simulink model "RoboCupManipulation_Simulink_ROS_Control"  (R2020b)
settings: Solver=FixedStepAuto  StartTime=0.0  StopTime=15  FixedStep=0.1  RelTol=1e-3
PreLoadFcn:
  | load('exampleHelperKINOVAGen3GripperROSGazebo.mat');
model workspace (MAT data in the model file):
  SL_ROS_VariableLengthArrays_MaxSizes.CommonInfo.ArrayTruncateAction = 'EmitWarning'
  SL_ROS_VariableLengthArrays_MaxSizes.MsgTypeMap = containers.Map
  SL_ROS_VariableLengthArrays_MaxSizes.MsgTypeMap.serialization.keys = {'sensor_msgs/Image'}
  SL_ROS_VariableLengthArrays_MaxSizes.MsgTypeMap.serialization.values{1}(1).PropertyName = 'Data'
  SL_ROS_VariableLengthArrays_MaxSizes.MsgTypeMap.serialization.values{1}(1).DataType = 'uint8'
  SL_ROS_VariableLengthArrays_MaxSizes.MsgTypeMap.serialization.values{1}(1).MaxLength = 518400
  SL_ROS_VariableLengthArrays_MaxSizes.MsgTypeMap.serialization.values{1}(2).PropertyName = 'Encoding'
  SL_ROS_VariableLengthArrays_MaxSizes.MsgTypeMap.serialization.values{1}(2).DataType = 'uint8'
  SL_ROS_VariableLengthArrays_MaxSizes.MsgTypeMap.serialization.values{1}(2).MaxLength = 128
  SL_ROS_VariableLengthArrays_MaxSizes.MsgTypeMap.serialization.uniformity = 0
  SL_ROS_VariableLengthArrays_MaxSizes.MsgTypeMap.serialization.keyType = 'char'
  SL_ROS_VariableLengthArrays_MaxSizes.MsgTypeMap.serialization.valueType = 'any'
undefined symbols (not defined in the file or in its folder): Angle, Axis, eul2tform, trvec2tform
libraries: robotlib x7, robotcorelib x5, robotmaniplib x2, robotgazebolib x1, simulink x1
settings Model: PacingRate=0.220000  Creator=amavromm  LastModifiedBy=josea
settings OptimizationCC: EnhancedBackFolding=on  PassReuseOutputArgsAs=Individual arguments  ZeroExternalMemoryAtStartup=off  ZeroInternalMemoryAtStartup=off  MaxStackSize=64  OptimizeBlockOrder=speed  DifferentSizesBufferReuse=on  OptimizationCustomize=off  EfficientTunableParamExpr=on
settings DebuggingCC: ParameterTunabilityLossMsg=error
settings HardwareCC: ProdBitPerPointer=32  ProdBitPerSizeT=32  ProdBitPerPtrDiffT=32  ProdLargestAtomicFloat=None  ProdIntDivRoundTo=Undefined  ProdEndianess=Unspecified  ProdWordSize=32  ProdHWDeviceType=Generic->Unspecified (assume 32-bit Generic)
settings SFSimCC: MATLABDynamicMemAlloc=off  SimTargetLang=C++
settings RTWCC: Description=Embedded Coder  SystemTargetFile=ert.tlc  HardwareBoard=Robot Operating System (ROS)  TLCOptions="-aInlineSetEventsForThisBaseRateFcn=TLC_FALSE -aSuppressMultiTaskScheduler=TLC_FALSE  -aRateBasedStepFcn=0"  TemplateMakefile=ert_default_tmf  Toolchain=Catkin  TargetLang=C++
settings CodeAppCC: ForceParamTrailComments=on  IgnoreCustomStorageClasses=off  OperatorAnnotations=on  SimulinkDataObjDesc=on  SFDataObjDesc=on  InsertBlockDesc=on

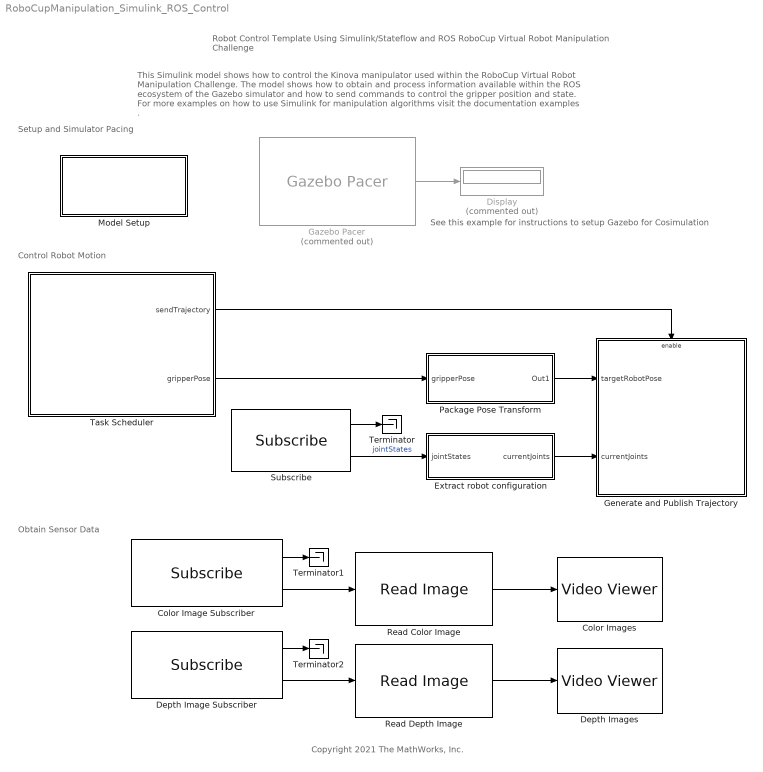
== system RoboCupManipulation_Simulink_ROS_Control ==
  note: See this example for instructions to setup Gazebo for Cosimulation
  note: This Simulink model shows how to control the Kinova manipulator used within the RoboCup Virtual Robot Manipulation Challenge. The model shows how to obtain and process information available within the ROS ecosystem of the Gazebo simulator and how to send commands to control the gripper position and state. For more examples on how to use Simulink for manipulation algorithms visit the documentation examples .
  note: Robot Control Template Using Simulink/Stateflow and ROS
      | RoboCup Virtual Robot Manipulation Challenge
  note: Obtain Sensor Data
  note: Control Robot Motion
  note: Setup and Simulator Pacing
  note: Copyright 2021 The MathWorks, Inc.
  Color Image Subscriber : robotlib/Subscribe  topicSource=Select from ROS network  topic=/camera/color/image_raw  messageType=sensor_msgs/Image  SampleTime=0.5  legacyBusStruct=off  messageQueueLength=1
  Color Images : VideoViewer  FigPos=[757 790 418 304]
  Depth Image Subscriber : robotlib/Subscribe  topicSource=Select from ROS network  topic=/camera/depth/image_raw  messageType=sensor_msgs/Image  SampleTime=0.5  legacyBusStruct=off  messageQueueLength=1
  Depth Images : VideoViewer  FigPos=[241 742 418 304]
  Display : Display  Commented=on
  Extract robot configuration : Subsystem
  Gazebo Pacer : robotgazebolib/Gazebo Pacer  Commented=on  ResetBehavior=Reset Gazebo simulation time  SampleTime=0.1
      settings: SourceProductBaseCode=RO
  Generate and Publish Trajectory : Subsystem
  Model Setup : Subsystem
  Package Pose Transform : Subsystem
  Read Color Image : robotlib/Read Image  MaximumImageSize=[270, 480]  ImageEncoding=rgb8  ShowAlphaOutput=off  ShowErrorCodeOutput=off  VariableSizeOutputs=off
      settings: SourceProductBaseCode=RR
  Read Depth Image : robotlib/Read Image  MaximumImageSize=[270, 480]  ImageEncoding=32fc1  ShowAlphaOutput=off  ShowErrorCodeOutput=off  VariableSizeOutputs=off
      settings: SourceProductBaseCode=RR
  Subscribe : robotlib/Subscribe  topicSource=Select from ROS network  topic=/my_gen3/joint_states  messageType=sensor_msgs/JointState  SampleTime=-1  legacyBusStruct=off  messageQueueLength=1
  Task Scheduler : Stateflow chart  TreatAsAtomicUnit=on
  Terminator : Terminator
  Terminator1 : Terminator
  Terminator2 : Terminator
  wires:
  Extract robot configuration/1(currentJoints) -> Generate and Publish Trajectory/2(currentJoints)
  Subscribe/2 -> Extract robot configuration/1(jointStates)  "jointStates"
  Task Scheduler/2(gripperPose) -> Package Pose Transform/1(gripperPose)
  Task Scheduler/1(sendTrajectory) -> Generate and Publish Trajectory/Enable
  Package Pose Transform/1(Out1) -> Generate and Publish Trajectory/1(targetRobotPose)
  Gazebo Pacer/1 -> Display/1
  Color Image Subscriber/2 -> Read Color Image/1
  Subscribe/1 -> Terminator/1
  Color Image Subscriber/1 -> Terminator1/1
  Read Color Image/1 -> Color Images/1
  Depth Image Subscriber/2 -> Read Depth Image/1
  Read Depth Image/1 -> Depth Images/1
  Depth Image Subscriber/1 -> Terminator2/1

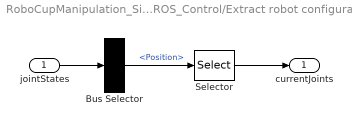
== system RoboCupManipulation_Simulink_ROS_Control/Extract robot configuration ==
  jointStates : Inport
  Bus Selector : BusSelector  OutputSignals=Position
  Selector : Selector  InputPortWidth=128  IndexOptions=Index vector (dialog)  Indices=[2:8]  OutputSizes=1
  currentJoints : Outport
  wires:
  Bus Selector/1 -> Selector/1  "<Position>"
  Selector/1 -> currentJoints/1
  jointStates/1 -> Bus Selector/1

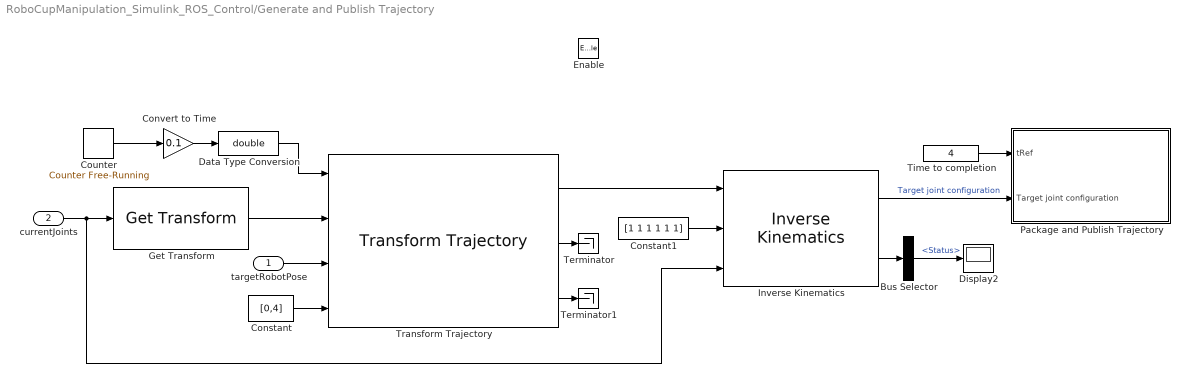
== system RoboCupManipulation_Simulink_ROS_Control/Generate and Publish Trajectory ==
  targetRobotPose : Inport
  currentJoints : Inport  Port=2
  Enable : EnablePort
  Bus Selector : BusSelector  OutputSignals=Status
  Constant : Constant  Value=[0,4]
  Constant1 : Constant  Value=[1 1 1 1 1 1]
  Convert to Time : Gain  Gain=0.1
  "Counter " : simulink/Sources/Counter Free-Running  NumBits=16  tsamp=0.1
  Data Type Conversion : DataTypeConversion  OutDataTypeStr=double
  Display2 : Display
  Get Transform : robotmaniplib/Get Transform  RigidBodyTree=robot  SourceBody=gripper  TargetBody=base_link  SimulateUsing=Interpreted execution
  Inverse Kinematics : robotmaniplib/Inverse Kinematics  RigidBodyTree=robot  EndEffector=gripper  ShowInfo=on  SolverName=BFGS Gradient Projection  EnforceJointLimits=on  MaxIterations=1500  MaxTime=10  GradientTolerance=1e-7  SolutionTolerance=1e-6  StepTolerance=1e-14  ErrorChangeTolerance=1e-12  UseErrorDamping=on  DampingBias=0.0025  SimulateUsing=Interpreted execution
  Package and Publish Trajectory : Subsystem
  Terminator : Terminator
  Terminator1 : Terminator
  Time to completion : Constant  Value=4
  Transform Trajectory : robotcorelib/Transform Trajectory  WaypointSource=External  T0=trvec2tform( [ 1, 10, -1 ] )  TF=eul2tform( [ 0, pi, pi / 2 ] )  TimeInterval=[ 2, 3 ]  CustomTimeScaling=off  ParameterSource=Internal  TSTime=2:0.1:3  TimeScaling=[ 0:0.1:1; ones( 1, 11 ); zeros( 1, 11 ) ]  SimulateUsing=Interpreted execution
      settings: SourceProductBaseCode=NV,RO,RR,UV
  wires:
  Constant1/1 -> Inverse Kinematics/2
  Transform Trajectory/1 -> Inverse Kinematics/1
  Constant/1 -> Transform Trajectory/4
  targetRobotPose/1 -> Transform Trajectory/3
  currentJoints/1 -> Inverse Kinematics/3, Get Transform/1
  Convert to Time/1 -> Data Type Conversion/1
  "Counter "/1 -> Convert to Time/1
  Data Type Conversion/1 -> Transform Trajectory/1
  Get Transform/1 -> Transform Trajectory/2
  Inverse Kinematics/2 -> Bus Selector/1
  Bus Selector/1 -> Display2/1  "<Status>"
  Time to completion/1 -> Package and Publish Trajectory/1(tRef)
  Inverse Kinematics/1 -> Package and Publish Trajectory/2(Target joint configuration)  "Target joint configuration"
  Transform Trajectory/2 -> Terminator/1
  Transform Trajectory/3 -> Terminator1/1

== system RoboCupManipulation_Simulink_ROS_Control/Model Setup ==
  note: 1
  note: Before running the Simulink model, make sure the ROS network requirements have been set appropriately through the Simulink Toolstrip and MATLAB ROS Node has been initiated. Note that setting a Node Host IP address is optional and depends on the computer setup.
  note: ROS Model Setup
  note: 22
  note: 23

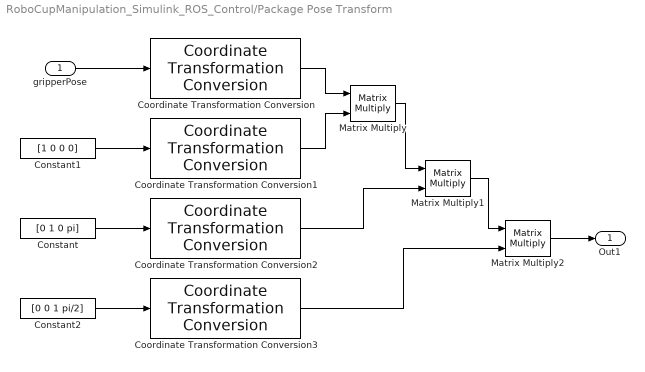
== system RoboCupManipulation_Simulink_ROS_Control/Package Pose Transform ==
  gripperPose : Inport
  Constant : Constant  Value=[0 1 0 pi]
  Constant1 : Constant  Value=[1 0 0 0]
  Constant2 : Constant  Value=[0 0 1 pi/2]
  Coordinate Transformation Conversion : robotcorelib/Coordinate Transformation Conversion  InputRepresentation=Translation Vector  InputEulerSequence=ZYX  ShowTrVecInputPort=on  OutputRepresentation=Homogeneous Transformation  OutputEulerSequence=ZYX  ShowTrVecOutputPort=on  SimulateUsing=Interpreted execution
      settings: SourceProductBaseCode=NV,RO,RR,UV
  Coordinate Transformation Conversion1 : robotcorelib/Coordinate Transformation Conversion  InputRepresentation=Axis-Angle  InputEulerSequence=ZYX  ShowTrVecInputPort=off  OutputRepresentation=Homogeneous Transformation  OutputEulerSequence=ZYX  ShowTrVecOutputPort=on  SimulateUsing=Interpreted execution
      settings: SourceProductBaseCode=NV,RO,RR,UV
  Coordinate Transformation Conversion2 : robotcorelib/Coordinate Transformation Conversion  InputRepresentation=Axis-Angle  InputEulerSequence=ZYX  ShowTrVecInputPort=off  OutputRepresentation=Homogeneous Transformation  OutputEulerSequence=ZYX  ShowTrVecOutputPort=on  SimulateUsing=Interpreted execution
      settings: SourceProductBaseCode=NV,RO,RR,UV
  Coordinate Transformation Conversion3 : robotcorelib/Coordinate Transformation Conversion  InputRepresentation=Axis-Angle  InputEulerSequence=ZYX  ShowTrVecInputPort=off  OutputRepresentation=Homogeneous Transformation  OutputEulerSequence=ZYX  ShowTrVecOutputPort=on  SimulateUsing=Interpreted execution
      settings: SourceProductBaseCode=NV,RO,RR,UV
  Matrix Multiply : Product  Multiplication=Matrix(*)
  Matrix Multiply1 : Product  Multiplication=Matrix(*)
  Matrix Multiply2 : Product  Multiplication=Matrix(*)
  Out1 : Outport
  wires:
  gripperPose/1 -> Coordinate Transformation Conversion/1
  Constant1/1 -> Coordinate Transformation Conversion1/1
  Constant2/1 -> Coordinate Transformation Conversion3/1
  Constant/1 -> Coordinate Transformation Conversion2/1
  Coordinate Transformation Conversion/1 -> Matrix Multiply/1
  Coordinate Transformation Conversion1/1 -> Matrix Multiply/2
  Matrix Multiply/1 -> Matrix Multiply1/1
  Coordinate Transformation Conversion2/1 -> Matrix Multiply1/2
  Matrix Multiply1/1 -> Matrix Multiply2/1
  Coordinate Transformation Conversion3/1 -> Matrix Multiply2/2
  Matrix Multiply2/1 -> Out1/1

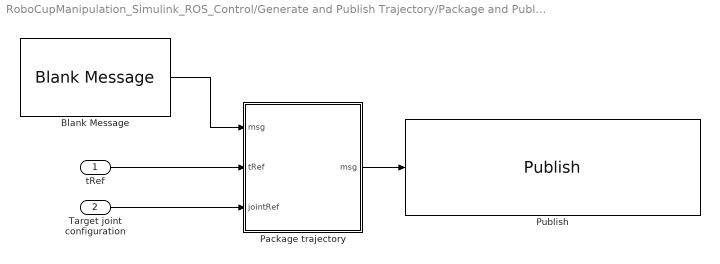
== system RoboCupManipulation_Simulink_ROS_Control/Generate and Publish Trajectory/Package and Publish Trajectory ==
  tRef : Inport
  Target joint configuration : Inport  Port=2
  Blank Message : robotlib/Blank Message  messageClass=Message  entityType=trajectory_msgs/JointTrajectory  messageType=trajectory_msgs/JointTrajectory  SampleTime=inf  legacyBusStruct=off
  Package trajectory : MATLAB Function  TreatAsAtomicUnit=on
  Publish : robotlib/Publish  topicSource=Select from ROS network  topic=/my_gen3/gen3_joint_trajectory_controller/command  messageType=trajectory_msgs/JointTrajectory  legacyBusStruct=off  messageQueueLength=1
  wires:
  Blank Message/1 -> Package trajectory/1("msg ")
  Package trajectory/1(msg) -> Publish/1
  Target joint configuration/1 -> Package trajectory/3(jointRef)
  tRef/1 -> Package trajectory/2(tRef)

== matlab function RoboCupManipulation_Simulink_ROS_Control/Generate and Publish Trajectory/Package and Publish Trajectory/Package trajectory ==
  data: msg input SL_Bus_RoboCupManipulation_Simul_JointTrajectory_eng8hf; msg output; tRef input; jointRef input
function msg = packageTrajectory(msg,tRef,jointRef)

    % Package joint names
    jointNames = {'joint_1','joint_2','joint_3','joint_4','joint_5','joint_6','joint_7'};
    numJoints = uint32(numel(jointNames));

    msg.JointNames_SL_Info.CurrentLength = uint32(7);
    for idx = 1:numJoints
       msg.JointNames(idx).Data(1:7) = uint8(jointNames{idx});
       msg.JointNames(idx).Data_SL_Info.CurrentLength = uint32(numJoints);
    end

    % Send next trajectory point
    msg.Points_SL_Info.CurrentLength = uint32(1);

    msg.Points(1).TimeFromStart.Sec = floor(tRef);
    msg.Points(1).TimeFromStart.Nsec = (tRef - floor(tRef))*1e9;

    msg.Points(1).Positions_SL_Info.CurrentLength = numJoints;
    msg.Points(1).Positions(1:numJoints) = jointRef;
    msg.Points(1).Velocities_SL_Info.CurrentLength = numJoints;
    msg.Points(1).Velocities(1:numJoints) = zeros(numJoints,1);
    msg.Points(1).Accelerations_SL_Info.CurrentLength = numJoints;
    msg.Points(1).Accelerations(1:numJoints) = zeros(numJoints,1);
    msg.Points(1).Effort_SL_Info.CurrentLength = numJoints;
    msg.Points(1).Effort(1:numJoints) = zeros(numJoints,1);

end

== stateflow chart RoboCupManipulation_Simulink_ROS_Control/Task Scheduler ==
  state Initialize
    gripperPose = [0.26 0 0.14]';
    sendTrajectory = 0;
    activateGripper(0);
  state MoveForward
    entry:
    gripperPose = [0.46 0 0.14]';
    during:
    sendTrajectory =1;
  state CloseGripper
    activateGripper(1);
  state MoveBackward
    entry:
    gripperPose = [0.26 0 0.14]';
    during:
    sendTrajectory = 1;
  state Idle
  (default) -> Initialize : {activateGripper(2);}
      | % Initialize Gripper Action Client
  Initialize -> MoveForward : [after(5,sec)]
  MoveForward -> CloseGripper : [after(4,sec)] {sendTrajectory=0;}
      | % Wait for trajectory following controller and disable
  CloseGripper -> MoveBackward
  MoveBackward -> Idle : [after(4,sec)] {sendTrajectory=0;}
  data: state function_input; sendTrajectory output; gripperPose output
  function activateGripper(state):
    | function activateGripper(state)
    |   coder.extrinsic('SLActivateGripper')
    |   SLActivateGripper(state)
    | end
